simulink model "Week3Problem1"  (R2020a)
settings: Solver=VariableStepAuto  StartTime=0.0  StopTime=10.0  RelTol=1e-3
settings Model: Creator=sreeram  LastModifiedBy=sreeram

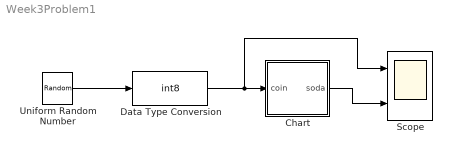
== system Week3Problem1 ==
  Chart : Stateflow chart  TreatAsAtomicUnit=on
  Data Type Conversion : DataTypeConversion  OutDataTypeStr=int8  RndMeth=Nearest  SaturateOnIntegerOverflow=on
  Scope : Scope  NumInputPorts=2
  Uniform Random Number : UniformRandomNumber  Minimum=0  Maximum=2  Seed=337  SampleTime=10
  wires:
  Uniform Random Number/1 -> Data Type Conversion/1
  Data Type Conversion/1 -> Scope/1, Chart/1(coin)
  Chart/1(soda) -> Scope/2

== stateflow chart Week3Problem1/Chart ==
  state got_0
  state got_nickel
  state got_dime
  (default) -> got_0
  got_0 -> got_nickel [order 1]
  got_nickel -> got_0 [order 2]
  got_dime -> got_0 [order 1]
  got_0 -> got_dime [order 2]
  got_nickel -> got_dime [order 1]
  got_dime -> got_nickel [order 2]
  data: coin input; soda output
